simulink model "plant_model"  (R2022a)
settings: Solver=VariableStepAuto  StartTime=0.0  StopTime=50  RelTol=1e-3
libraries: spsStairGeneratorLib x2
settings Model: Creator=ritvi  LastModifiedBy=ritvi

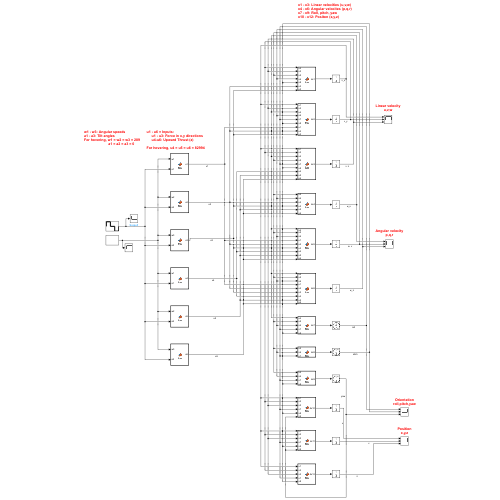
[thumbnail: Simulink's stored preview of the top-level diagram]
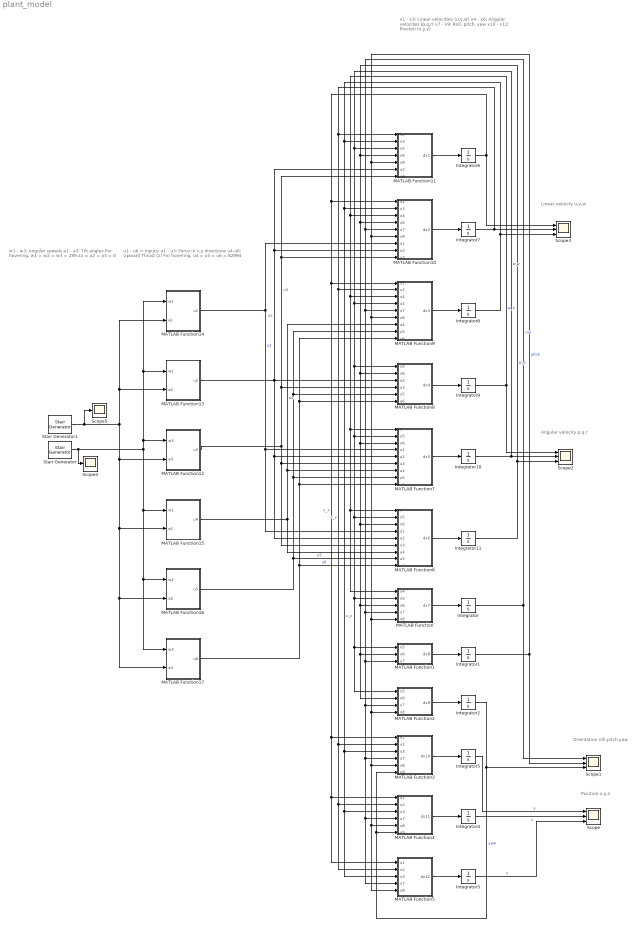
== system plant_model ==
  note: u1 - u6 = Inputs:
      | u1 - u3: Force in x,y directions
      | u4-u6: Upward Thrust (z)
      |
      | For hovering, u4 = u5 = u6 = 82994
  note: x1 - x3: Linear velocities (u,v,w)
      | x4 - x6: Angular velocites (p,q,r)
      | x7 - x9: Roll, pitch, yaw
      | x10 - x12: Positon (x,y,z)
  note: Orientation
      | roll,pitch,yaw
  note: Position
      | x,y,z
  note: w1 - w3: Angular speeds
      | a1 - a3: Tilt angles
      | For hovering, w1 = w2 = w3 = 289
      | a1 = a2 = a3 = 0
  note: Angular velocity
      | p,q,r
  note: Linear velocity
      | u,v,w
  Integrator : Integrator  WrapState=on
  Integrator1 : Integrator  WrapState=on
  Integrator{4..11} (8 alike) : Integrator
  Integrator2 : Integrator  WrapState=on
  Integrator3 : Integrator  LowerSaturationLimit=0
  MATLAB Function : MATLAB Function  TreatAsAtomicUnit=on
  MATLAB Function1 : MATLAB Function  TreatAsAtomicUnit=on
  MATLAB Function10 : MATLAB Function  TreatAsAtomicUnit=on
  MATLAB Function11 : MATLAB Function  TreatAsAtomicUnit=on
  MATLAB Function12 : MATLAB Function  TreatAsAtomicUnit=on
  MATLAB Function13 : MATLAB Function  TreatAsAtomicUnit=on
  MATLAB Function14 : MATLAB Function  TreatAsAtomicUnit=on
  MATLAB Function15 : MATLAB Function  TreatAsAtomicUnit=on
  MATLAB Function16 : MATLAB Function  TreatAsAtomicUnit=on
  MATLAB Function17 : MATLAB Function  TreatAsAtomicUnit=on
  MATLAB Function2 : MATLAB Function  TreatAsAtomicUnit=on
  MATLAB Function3 : MATLAB Function  TreatAsAtomicUnit=on
  MATLAB Function4 : MATLAB Function  TreatAsAtomicUnit=on
  MATLAB Function5 : MATLAB Function  TreatAsAtomicUnit=on
  MATLAB Function6 : MATLAB Function  TreatAsAtomicUnit=on
  MATLAB Function7 : MATLAB Function  TreatAsAtomicUnit=on
  MATLAB Function8 : MATLAB Function  TreatAsAtomicUnit=on
  MATLAB Function9 : MATLAB Function  TreatAsAtomicUnit=on
  Scope{,1..3} (4 alike) : Scope  NumInputPorts=3
  Scope4 : Scope
  Scope5 : Scope
  Stair Generator : spsStairGeneratorLib/Stair Generator  t=[0]  e=[300]  Ts=0
  Stair Generator1 : spsStairGeneratorLib/Stair Generator  t=[0, 2, 4,6,8]  e=[0,0.1,0,-0.1,0]  Ts=0
  wires:
  MATLAB Function5/1(dx12) -> Integrator3/1
  MATLAB Function4/1(dx11) -> Integrator4/1
  MATLAB Function3/1(dx10) -> Integrator5/1
  MATLAB Function2/1(dx9) -> Integrator2/1
  MATLAB Function1/1(dx8) -> Integrator1/1
  MATLAB Function/1(dx7) -> Integrator/1
  MATLAB Function11/1(dx1) -> Integrator6/1
  MATLAB Function10/1(dx2) -> Integrator7/1
  MATLAB Function9/1(dx3) -> Integrator8/1
  MATLAB Function8/1(dx4) -> Integrator9/1
  MATLAB Function7/1(dx5) -> Integrator10/1
  MATLAB Function6/1(dx6) -> Integrator11/1
  Integrator6/1 -> MATLAB Function5/1(x1), MATLAB Function4/1(x1), MATLAB Function3/1(x1), MATLAB Function9/1(x1), MATLAB Function10/1(x1), Scope3/1  "v_x"
  Integrator7/1 -> Scope3/2, MATLAB Function5/2(x2), MATLAB Function4/2(x2), MATLAB Function3/2(x2), MATLAB Function9/2(x2), MATLAB Function11/1(x2)  "v_y"
  Integrator8/1 -> Scope3/3, MATLAB Function5/3(x3), MATLAB Function4/3(x3), MATLAB Function3/3(x3), MATLAB Function10/2(x3), MATLAB Function11/2(x3)  "v_z"
  Integrator9/1 -> MATLAB Function/1(x4), MATLAB Function6/1(x4), MATLAB Function7/1(x4), MATLAB Function9/3(x4), MATLAB Function10/3(x4), Scope2/1  "w_x"
  Integrator10/1 -> Scope2/2, MATLAB Function2/1(x5), MATLAB Function1/1(x5), MATLAB Function/2(x5), MATLAB Function6/2(x5), MATLAB Function7/2(x5), MATLAB Function8/1(x5), MATLAB Function9/4(x5), MATLAB Function11/3(x5)  "w_y"
  Integrator11/1 -> Scope2/3, MATLAB Function2/2(x6), MATLAB Function1/2(x6), MATLAB Function/3(x6), MATLAB Function6/3(x6), MATLAB Function7/3(x6), MATLAB Function8/2(x6), MATLAB Function10/4(x6), MATLAB Function11/4(x6)  "w_z"
  Integrator/1 -> Scope1/1, MATLAB Function5/4(x7), MATLAB Function4/4(x7), MATLAB Function3/4(x7), MATLAB Function2/3(x7), MATLAB Function1/3(x7), MATLAB Function/4(x7), MATLAB Function9/5(x7), MATLAB Function10/5(x7)  "roll"
  Integrator1/1 -> Scope1/2, MATLAB Function2/4(x8), MATLAB Function5/5(x8), MATLAB Function4/5(x8), MATLAB Function3/5(x8), MATLAB Function/5(x8), MATLAB Function9/6(x8), MATLAB Function10/6(x8), MATLAB Function11/5(x8)  "pitch"
  Integrator2/1 -> MATLAB Function4/6(x9), MATLAB Function3/6(x9), Scope1/3  "yaw"
  MATLAB Function14/1(u1) -> MATLAB Function6/4(u1), MATLAB Function7/4(u1), MATLAB Function10/7(u1)  "u1"
  MATLAB Function13/1(u2) -> MATLAB Function8/3(u2), MATLAB Function10/8(u2), MATLAB Function11/6(u2), MATLAB Function7/5(u2), MATLAB Function6/5(u2)  "u2"
  MATLAB Function12/1(u3) -> MATLAB Function7/6(u3), MATLAB Function6/6(u3), MATLAB Function8/4(u3), MATLAB Function10/9(u3), MATLAB Function11/7(u3)  "u3"
  MATLAB Function15/1(u4) -> MATLAB Function6/7(u4), MATLAB Function7/7(u4), MATLAB Function9/7(u4)  "u4"
  MATLAB Function16/1(u5) -> MATLAB Function6/8(u5), MATLAB Function7/8(u5), MATLAB Function8/5(u5), MATLAB Function9/8(u5)  "u5"
  MATLAB Function17/1(u6) -> MATLAB Function6/9(u6), MATLAB Function7/9(u6), MATLAB Function8/6(u6), MATLAB Function9/9(u6)  "u6"
  Integrator3/1 -> Scope/3  "z"
  Integrator4/1 -> Scope/2  "y"
  Integrator5/1 -> Scope/1  "x"
  Stair Generator1/1 -> Scope5/1, MATLAB Function13/2(a2), MATLAB Function14/2(a1), MATLAB Function17/2(a3), MATLAB Function16/2(a2), MATLAB Function15/2(a1), MATLAB Function12/2(a3)
  Stair Generator/1 -> Scope4/1, MATLAB Function15/1(w1), MATLAB Function16/1(w2), MATLAB Function17/1(w3), MATLAB Function12/1(w3), MATLAB Function13/1(w2), MATLAB Function14/1(w1)

== matlab function plant_model/MATLAB Function8 ==
  data: dx4 output; x5 input; x6 input; u2 input; u3 input; u5 input; u6 input
function dx4 = fcn(x5,x6,u2,u3,u5,u6)

m = 0.5;
g = 9.81;
l = 0.23;
Ixx = 6.8*10^-3;
Iyy = 5.3*10^-3;
Izz = 1.7*10^-3;
Iyz = 3.1*10^-4;
kf = 1.97*10^-5;
kd = 0.0; %2.88*10^-7;

dx4 = (x5*x6*(Iyy - Izz) + Iyz*(x5^2 - x6^2) + 0.5*sqrt(3)*kd*u2 - 0.5*sqrt(3)*kd*u3 + 0.5*sqrt(3)*l*kf*u5 - 0.5*sqrt(3)*l*kf*u6)/Ixx;

== matlab function plant_model/MATLAB Function9 ==
  data: x1 input; x2 input; x4 input; dx3 output; x5 input; x7 input; x8 input; u4 input; u5 input; u6 input
function dx3 = fcn(x1,x2,x4,x5,x7,x8,u4,u5,u6)

m = 0.5;
g = 9.81;
l = 0.23;
Ixx = 6.8*10^-3;
Iyy = 5.3*10^-3;
Izz = 1.7*10^-3;
Iyz = 3.1*10^-4;
kf = 1.97*10^-5;
kd = 2.88*10^-7;

dx3 = x1*x5 - x2*x4 - g*cos(x7)*cos(x8) + kf*u4/m + kf*u5/m + kf*u6/m;

== matlab function plant_model/MATLAB Function10 ==
  data: x1 input; x3 input; x4 input; dx2 output; x6 input; x7 input; x8 input; u1 input; u2 input; u3 input
function dx2 = fcn(x1,x3,x4,x6,x7,x8,u1,u2,u3)

m = 0.5;
g = 9.81;
l = 0.23;
Ixx = 6.8*10^-3;
Iyy = 5.3*10^-3;
Izz = 1.7*10^-3;
Iyz = 3.1*10^-4;
kf = 1.97*10^-5;
kd = 2.88*10^-7;

dx2 = x3*x4 - x1*x6 - g*sin(x7)*cos(x8) + kf*u1/m - 0.5*kf*u2/m - 0.5*kf*u3/m;

== matlab function plant_model/MATLAB Function11 ==
  data: x2 input; x3 input; x5 input; dx1 output; x6 input; x8 input; u2 input; u3 input
function dx1 = fcn(x2,x3,x5,x6,x8,u2,u3)

m = 0.5;
g = 9.81;
l = 0.23;
Ixx = 6.8*10^-3;
Iyy = 5.3*10^-3;
Izz = 1.7*10^-3;
Iyz = 3.1*10^-4;
kf = 1.97*10^-5;
kd = 2.88*10^-7;

dx1 = x2*x6 - x3*x5 + g*sin(x8) - 0.5*sqrt(3)*kf*u2/m + 0.5*sqrt(3)*kf*u3/m;

== matlab function plant_model/MATLAB Function12 ==
  data: u3 output; w3 input; a3 input
function u3 = fcn(w3,a3)

u3 = (w3^2)*sin(a3);

== matlab function plant_model/MATLAB Function13 ==
  data: u2 output; w2 input; a2 input
function u2 = fcn(w2,a2)

u2 = (w2^2)*sin(a2);

== matlab function plant_model/MATLAB Function1 ==
  data: dx8 output; x5 input; x6 input; x7 input
function dx8 = fcn(x5,x6,x7)

dx8 = x5*cos(x7) - x6*sin(x7);

== matlab function plant_model/MATLAB Function14 ==
  data: u1 output; w1 input; a1 input
function u1 = fcn(w1,a1)

u1 = (w1^2)*sin(a1);

== matlab function plant_model/MATLAB Function15 ==
  data: u4 output; w1 input; a1 input
function u4 = fcn(w1,a1)

u4 = (w1^2)*cos(a1);

== matlab function plant_model/MATLAB Function16 ==
  data: u5 output; w2 input; a2 input
function u5 = fcn(w2,a2)

u5 = (w2^2)*cos(a2);

== matlab function plant_model/MATLAB Function17 ==
  data: u6 output; w3 input; a3 input
function u6 = fcn(w3,a3)

u6 = (w3^2)*cos(a3);

== matlab function plant_model/MATLAB Function ==
  data: x4 input; dx7 output; x5 input; x6 input; x7 input; x8 input
function dx7 = fcn(x4,x5,x6,x7,x8)

dx7 = x4 + x5*sin(x7)*tan(x8) + x6*cos(x7)*tan(x8);

== matlab function plant_model/MATLAB Function2 ==
  data: dx9 output; x5 input; x6 input; x7 input; x8 input
function dx9 = fcn(x5,x6,x7,x8)

dx9 = x5*sin(x7)*sec(x8) + x6*cos(x7)*sec(x8);

== matlab function plant_model/MATLAB Function3 ==
  data: x1 input; x2 input; x3 input; dx10 output; x7 input; x8 input; x9 input
function dx10 = fcn(x1,x2,x3,x7,x8,x9)

dx10 = x1*cos(x8)*cos(x9) + x2*(sin(x7)*sin(x8)*cos(x9) - cos(x7)*sin(x9)) + x3*(cos(x7)*sin(x8)*cos(x9) + sin(x7)*sin(x9));

== matlab function plant_model/MATLAB Function4 ==
  data: x1 input; x2 input; x3 input; dx11 output; x7 input; x8 input; x9 input
function dx11 = fcn(x1,x2,x3,x7,x8,x9)

dx11 = x1*cos(x8)*sin(x9) + x2*(sin(x7)*sin(x8)*sin(x9) - cos(x7)*cos(x9)) + x3*(cos(x7)*sin(x8)*sin(x9) - sin(x7)*cos(x9));

== matlab function plant_model/MATLAB Function5 ==
  data: x1 input; x2 input; x3 input; dx12 output; x7 input; x8 input
function dx12 = fcn(x1,x2,x3,x7,x8)

dx12 = -x1*sin(x8) + x2*sin(x7)*cos(x8) + x3*cos(x7)*cos(x8);

== matlab function plant_model/MATLAB Function6 ==
  data: x4 input; dx6 output; x5 input; x6 input; u1 input; u2 input; u3 input; u4 input; u5 input; u6 input
function dx6 = fcn(x4,x5,x6,u1,u2,u3,u4,u5,u6)

m = 0.5;
g = 9.81;
l = 0.23;
Ixx = 6.8*10^-3;
Iyy = 5.3*10^-3;
Izz = 1.7*10^-3;
Iyz = 3.1*10^-4;
kf = 1.97*10^-5;
kd = 0.0; %2.88*10^-7;

dx6 = (x4*x6*(Iyy*Izz + Izz*Iyz - Ixx*Iyz) + x4*x5*(Ixx*Iyy - Iyz^2 - Iyy^2) + u1*(Iyy*kf*l - Iyz*kd) + u2*(Iyy*kf*l + 0.5*Iyz*kd) + u3*(Iyy*kf*l + 0.5*Iyz*kd) - u4*(Iyz*kf*l + Iyy*kd) + u5*(0.5*Iyz*kf*l - Iyy*kd) + u6*(0.5*Iyz*kf*l - Iyy*kd))/(Iyy*Izz - Iyz^2);

== matlab function plant_model/MATLAB Function7 ==
  data: x4 input; dx5 output; x5 input; x6 input; u1 input; u2 input; u3 input; u4 input; u5 input; u6 input
function dx5 = fcn(x4,x5,x6,u1,u2,u3,u4,u5,u6)

m = 0.5;
g = 9.81;
l = 0.23;
Ixx = 6.8*10^-3;
Iyy = 5.3*10^-3;
Izz = 1.7*10^-3;
Iyz = 3.1*10^-4;
kf = 1.97*10^-5;
kd = 0.0; %2.88*10^-7;

dx5 = (x4*x5*(Ixx*Iyz + Iyy*Iyz - Izz*Iyz) + x4*x6*(Iyz^2 + Izz^2 - Ixx*Izz) + u1*(Iyz*kf*l - Izz*kd) + u2*(Iyz*kf*l + 0.5*Izz*kd) + u3*(Iyz*kf*l + 0.5*Izz*kd) - u4*(Izz*kf*l + Iyz*kd) + u5*(0.5*Izz*kf*l - Iyz*kd) + u6*(0.5*Izz*kf*l - Iyz*kd))/(Iyy*Izz - Iyz^2);
